simulink model "openLoop"  (R2022a)
settings: Solver=FixedStepAuto  StartTime=0.0  StopTime=inf  FixedStep=0.01  RelTol=1e-3
undefined symbols (not defined in the file or in its folder): Levenberg, Marquardt, w, x, y, z
libraries: ros2lib x2, robotcorelib x1, robotmaniplib x1
settings Model: Creator=alessandrini  LastModifiedBy=alessandrini
settings SolverCC: AlgebraicLoopSolver=TrustRegion
settings OptimizationCC: EnhancedBackFolding=on  PassReuseOutputArgsAs=Individual arguments  ZeroExternalMemoryAtStartup=off  ZeroInternalMemoryAtStartup=off  MaxStackSize=64  OptimizeBlockOrder=speed  DifferentSizesBufferReuse=on  OptimizationCustomize=off  EfficientTunableParamExpr=on
settings DebuggingCC: ParameterTunabilityLossMsg=error  UnconnectedInputMsg=warning  UnconnectedOutputMsg=warning  UnconnectedLineMsg=warning  SFMachineParentedDataDiag=warning
settings HardwareCC: ProdBitPerLong=64  ProdHWDeviceType=Intel->x86-64 (Linux 64)  UseEmbeddedCoderFeatures=off
settings SFSimCC: MATLABDynamicMemAlloc=off
settings RTWCC: SystemTargetFile=ert.tlc  HardwareBoard=Robot Operating System 2 (ROS 2)  TLCOptions="-aInlineSetEventsForThisBaseRateFcn=TLC_FALSE -aSuppressMultiTaskScheduler=TLC_FALSE  -aRateBasedStepFcn=0"  TemplateMakefile=ert_default_tmf  Toolchain=Colcon Tools  TargetLang=C++  DLArmComputeVersion=19.05
settings CodeAppCC: ForceParamTrailComments=on  IgnoreCustomStorageClasses=off  OperatorAnnotations=on  SimulinkDataObjDesc=on  SFDataObjDesc=on  InsertBlockDesc=on
settings ERTTargetCC: CodeInterfacePackaging=C++ class  SupportNonInlinedSFcns=on  RootIOFormat=Structure reference

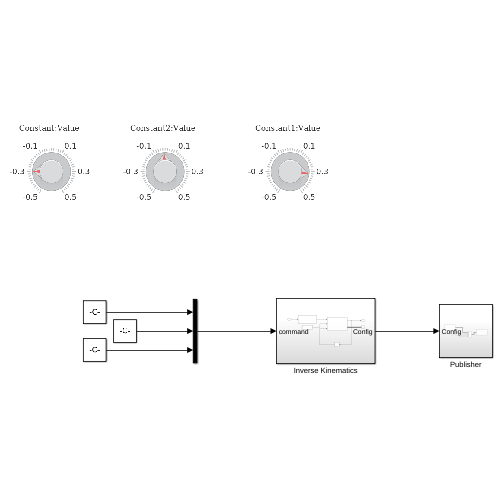
[thumbnail: Simulink's stored preview of the top-level diagram]
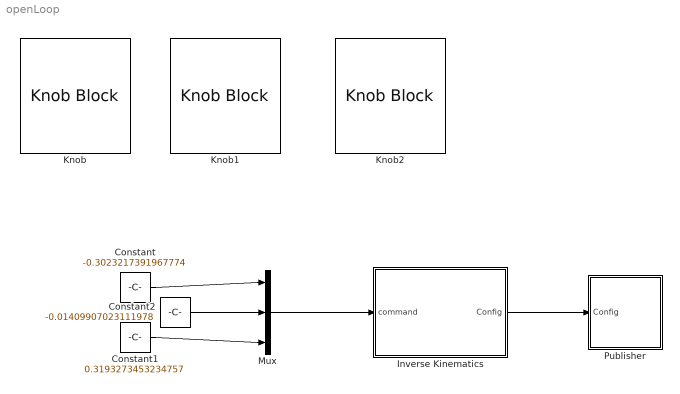
== system openLoop ==
  Constant : Constant  Value=-0.3023217391967774
  Constant1 : Constant  Value=0.3193273453234757
  Constant2 : Constant  Value=-0.01409907023111978
  Inverse Kinematics : Subsystem
  Knob : KnobBlock  ScaleMin=-0.5  ScaleMax=0.5
  Knob1 : KnobBlock  ScaleMin=-0.5  ScaleMax=0.5
  Knob2 : KnobBlock  ScaleMin=-0.5  ScaleMax=0.5
  Mux : Mux  Inputs=3
  Publisher : Subsystem
  wires:
  Mux/1 -> Inverse Kinematics/1(command)
  Inverse Kinematics/1(Config) -> Publisher/1(Config)
  Constant/1 -> Mux/1
  Constant1/1 -> Mux/3
  Constant2/1 -> Mux/2

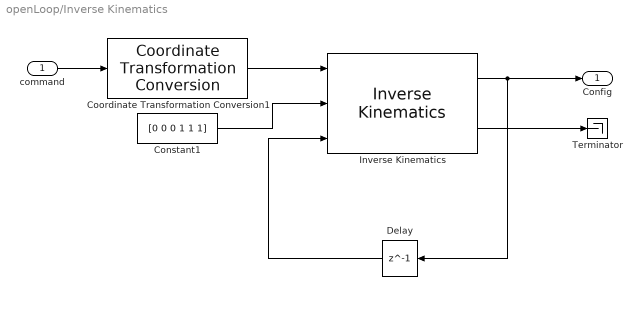
== system openLoop/Inverse Kinematics ==
  command : Inport
  Constant1 : Constant  Value=[0 0 0 1 1 1]  VectorParams1D=off
  Coordinate Transformation Conversion1 : robotcorelib/Coordinate Transformation Conversion  InputRepresentation=Translation Vector  InputEulerSequence=ZYX  ShowTrVecInputPort=on  OutputRepresentation=Homogeneous Transformation  OutputEulerSequence=ZYX  ShowTrVecOutputPort=on  SimulateUsing=Interpreted execution
  Delay : Delay  DelayLength=1  InitialCondition=([0 -10 0 90]*pi/180)'
  Inverse Kinematics : robotmaniplib/Inverse Kinematics  RigidBodyTree=robot  EndEffector=Body5  ShowInfo=on  SolverName=Levenberg-Marquardt  EnforceJointLimits=on  MaxIterations=1500  MaxTime=10  GradientTolerance=1e-7  SolutionTolerance=1e-6  StepTolerance=1e-14  ErrorChangeTolerance=1e-12  UseErrorDamping=on  DampingBias=0.0025  SimulateUsing=Interpreted execution
  Terminator : Terminator
  Config : Outport
  wires:
  Coordinate Transformation Conversion1/1 -> Inverse Kinematics/1
  Delay/1 -> Inverse Kinematics/3
  Constant1/1 -> Inverse Kinematics/2
  command/1 -> Coordinate Transformation Conversion1/1
  Inverse Kinematics/2 -> Terminator/1
  Inverse Kinematics/1 -> Config/1, Delay/1

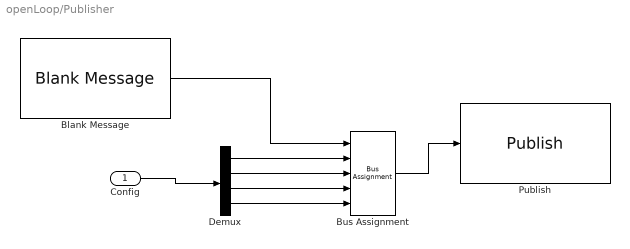
== system openLoop/Publisher ==
  Config : Inport
  Blank Message : ros2lib/Blank Message  messageClass=Message  entityType=geometry_msgs/Quaternion  messageType=geometry_msgs/Quaternion  SampleTime=0.01
      settings: SourceProductBaseCode=RR
  Bus Assignment : BusAssignment  AssignedSignals=x,y,z,w
  Demux : Demux
  Publish : ros2lib/Publish  topicSource=Specify your own  topic=/Command  messageType=geometry_msgs/Quaternion  QOSHistory=Keep last  QOSDepth=1  QOSReliability=Reliable  QOSDurability=Volatile
      settings: SourceProductBaseCode=RR
  wires:
  Blank Message/1 -> Bus Assignment/1
  Bus Assignment/1 -> Publish/1
  Config/1 -> Demux/1
  Demux/1 -> Bus Assignment/2
  Demux/2 -> Bus Assignment/3
  Demux/3 -> Bus Assignment/4
  Demux/4 -> Bus Assignment/5
